simulink model "Schema_Complet"  (R2015b)
settings: Solver=VariableStepAuto  StartTime=0.0  StopTime=5000  RelTol=1e-3
values from neighbouring files (symbols this model uses):
  k = 1/5    (= 0.2)    [constantes.m]
  Kc = 1.3    [constantes.m]
  Kcapt = 5*10^(-3)    (= 0.005)    [constantes.m]
  Km = 1/Ke    (= 0.769230769231)    [constantes.m]
  Kr = Rp*k    (= 0.009)    [constantes.m]
  L = 0.009    [constantes.m]
  R = 3    [constantes.m]
  Rp = 45*10^(-3)    (= 0.045)    [constantes.m]
  Te = (-b-sqrt(delta))/(2*a)    [constantes.m]
  Tm = (L*Jeq)/(Kc*Ke*te1)    [constantes.m]
settings Model: Creator=pt_ptsi  LastModifiedBy=pt_ptsi

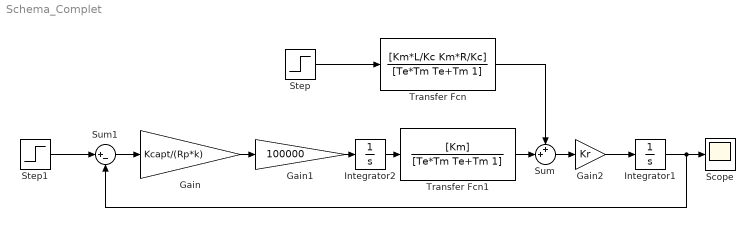
== system Schema_Complet ==
  Gain : Gain  Gain=Kcapt/(Rp*k)
  Gain1 : Gain  Gain=100000
  Gain2 : Gain  Gain=Kr
  Integrator1 : Integrator
  Integrator2 : Integrator
  Scope : Scope
  Step : Step  Time=0  SampleTime=0
  Step1 : Step  Time=0  SampleTime=0
  Sum : Sum  Inputs=++|
  Sum1 : Sum  Inputs=|+-
  Transfer Fcn : TransferFcn  Numerator=[Km*L/Kc Km*R/Kc]  Denominator=[Te*Tm Te+Tm 1]
  Transfer Fcn1 : TransferFcn  Numerator=[Km]  Denominator=[Te*Tm Te+Tm 1]
  wires:
  Transfer Fcn1/1 -> Sum/2
  Transfer Fcn/1 -> Sum/1
  Step/1 -> Transfer Fcn/1
  Step1/1 -> Sum1/1
  Sum1/1 -> Gain/1
  Gain/1 -> Gain1/1
  Sum/1 -> Gain2/1
  Gain2/1 -> Integrator1/1
  Integrator1/1 -> Sum1/2, Scope/1
  Gain1/1 -> Integrator2/1
  Integrator2/1 -> Transfer Fcn1/1
